simulink subsystem "proc_nav_ros_input"  (R2021a)
settings: Solver=VariableStepAuto  StartTime=0.0  StopTime=10.0  RelTol=1e-3
undefined symbols (not defined in the file): simulink
libraries: robotlib x6, simulink x2
settings Model: Creator=lamarre  LastModifiedBy=lamarre
settings SolverCC: AlgebraicLoopSolver=TrustRegion
settings DebuggingCC: SFMachineParentedDataDiag=warning

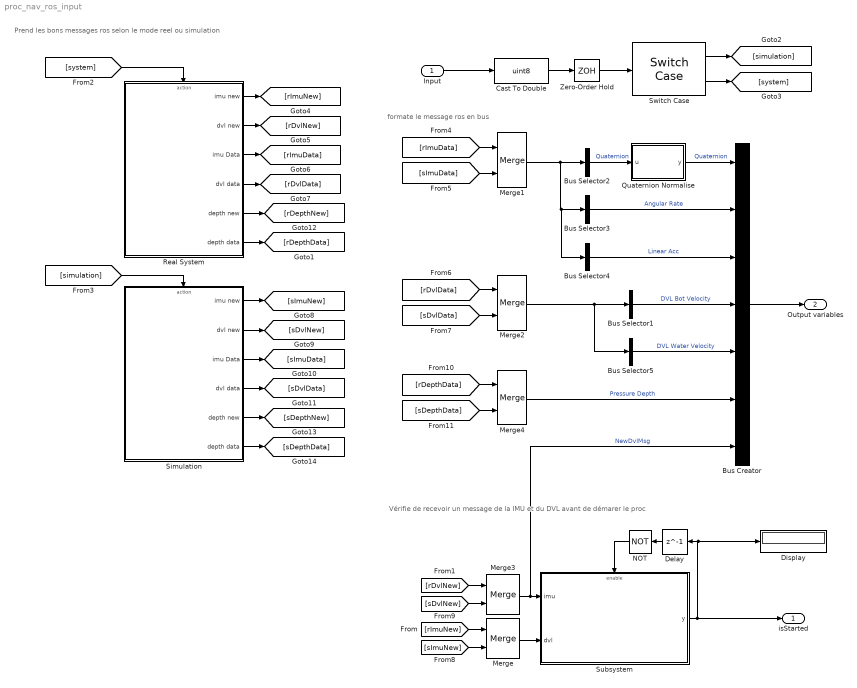
== system proc_nav_ros_input ==
  note: formate le message ros en bus
  note: Prend les bons messages ros selon le mode reel ou simulation
  note: Vérifie de recevoir un message de la IMU et
      |  du DVL avant de démarer le proc
  Input : Inport
  Bus Creator : BusCreator  Inputs=7
  Bus Selector1 : BusSelector  OutputSignals=XVelBtm,YVelBtm,ZVelBtm,EVelBtm  OutputAsBus=on
  Bus Selector2 : BusSelector  OutputSignals=Orientation.W,Orientation.X,Orientation.Y,Orientation.Z  OutputAsBus=on
  Bus Selector3 : BusSelector  OutputSignals=AngularVelocity  OutputAsBus=on
  Bus Selector4 : BusSelector  OutputSignals=LinearAcceleration  OutputAsBus=on
  Bus Selector5 : BusSelector  OutputSignals=Velocity1,Velocity2,Velocity3,Velocity4  OutputAsBus=on
  Cast To Double : DataTypeConversion  OutDataTypeStr=uint8
  Delay : Delay  DelayLength=1  InitialCondition=0
  Display : Display
  Merge{,1..4} (5 alike) : Merge
  NOT : Logic  Operator=NOT  AllPortsSameDT=off  OutDataTypeStr=boolean
  Quaternion Normalise : MATLAB Function  TreatAsAtomicUnit=on
  Real System : Subsystem  TreatAsAtomicUnit=on
  Simulation : Subsystem  TreatAsAtomicUnit=on
  Subsystem : Subsystem
  Switch Case : SwitchCase
  Zero-Order Hold : ZeroOrderHold  SampleTime=simulink.procNav.sampletime
  isStarted : Outport
  Output variables : Outport  Port=2
  wires:
  Bus Selector3/1 -> Bus Creator/2  "Angular Rate"
  Bus Selector1/1 -> Bus Creator/4  "DVL Bot Velocity"
  Bus Creator/1 -> Output variables/1
  Merge1/1 -> Bus Selector2/1, Bus Selector3/1, Bus Selector4/1
  Bus Selector2/1 -> Quaternion Normalise/1(u)  "Quaternion"
  Quaternion Normalise/1(y) -> Bus Creator/1  "Quaternion"
  Bus Selector4/1 -> Bus Creator/3  "Linear Acc"
  Bus Selector5/1 -> Bus Creator/5  "DVL Water Velocity"
  Switch Case/2 -> [system]
  Switch Case/1 -> [simulation]
  [system] -> Real System/Action
  [simulation] -> Simulation/Action
  Zero-Order Hold/1 -> Switch Case/1
  Input/1 -> Cast To Double/1
  Cast To Double/1 -> Zero-Order Hold/1
  Delay/1 -> NOT/1
  NOT/1 -> Subsystem/Enable
  Real System/1(imu new) -> [rImuNew]
  Simulation/4(dvl data) -> [sDvlData]
  Simulation/3(imu Data) -> [sImuData]
  Simulation/2(dvl new) -> [sDvlNew]
  Simulation/1(imu new) -> [sImuNew]
  Real System/4(dvl data) -> [rDvlData]
  Real System/3(imu Data) -> [rImuData]
  Real System/2(dvl new) -> [rDvlNew]
  [rImuData] -> Merge1/1
  [sImuData] -> Merge1/2
  [sDvlData] -> Merge2/2
  [rDvlData] -> Merge2/1
  [rImuNew] -> Merge/1
  [sImuNew] -> Merge/2
  [rDvlNew] -> Merge3/1
  [sDvlNew] -> Merge3/2
  Merge3/1 -> Bus Creator/7, Subsystem/1(imu)  "NewDvlMsg"
  Merge/1 -> Subsystem/2(dvl)
  Merge4/1 -> Bus Creator/6  "Pressure Depth"
  Real System/6(depth data) -> [rDepthData]
  Real System/5(depth new) -> [rDepthNew]
  Simulation/5(depth new) -> [sDepthNew]
  Simulation/6(depth data) -> [sDepthData]
  [sDepthData] -> Merge4/2
  [rDepthData] -> Merge4/1
  Subsystem/1(y) -> isStarted/1, Delay/1, Display/1
  Merge2/1 -> Bus Selector1/1, Bus Selector5/1

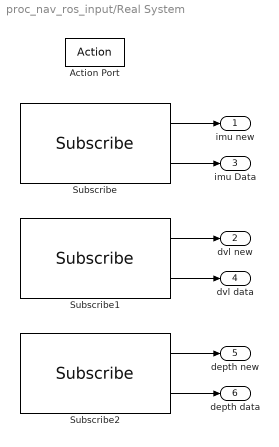
== system proc_nav_ros_input/Real System ==
  Action Port : ActionPort
  Subscribe : robotlib/Subscribe  topicSource=Specify your own  topic=/provider_imu/imu_info  messageType=sensor_msgs/Imu  SampleTime=simulink.procNav.sampletime  legacyBusStruct=off  messageQueueLength=1
  Subscribe1 : robotlib/Subscribe  topicSource=Specify your own  topic=/provider_dvl/dvl_velocity  messageType=sonia_common/BodyVelocityDVL  SampleTime=simulink.procNav.sampletime  legacyBusStruct=off  messageQueueLength=1
  Subscribe2 : robotlib/Subscribe  topicSource=Specify your own  topic=/provider_depth/depth  messageType=std_msgs/Float32  SampleTime=simulink.procNav.sampletime  legacyBusStruct=off  messageQueueLength=1
  imu new : Outport
  dvl new : Outport  Port=2
  imu Data : Outport  Port=3
  dvl data : Outport  Port=4
  depth new : Outport  Port=5
  depth data : Outport  Port=6
  wires:
  Subscribe2/1 -> depth new/1
  Subscribe2/2 -> depth data/1
  Subscribe/2 -> imu Data/1
  Subscribe1/1 -> dvl new/1
  Subscribe1/2 -> dvl data/1
  Subscribe/1 -> imu new/1

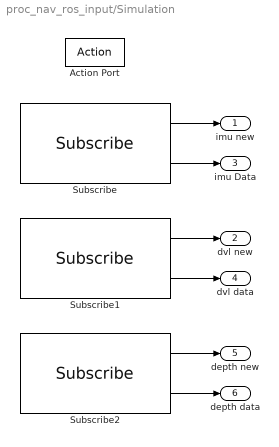
== system proc_nav_ros_input/Simulation ==
  Action Port : ActionPort
  Subscribe : robotlib/Subscribe  topicSource=Specify your own  topic=/proc_simulation/imu_info  messageType=sensor_msgs/Imu  SampleTime=simulink.procNav.sampletime  legacyBusStruct=off  messageQueueLength=1
  Subscribe1 : robotlib/Subscribe  topicSource=Specify your own  topic=/proc_simulation/dvl_velocity  messageType=sonia_common/BodyVelocityDVL  SampleTime=simulink.procNav.sampletime  legacyBusStruct=off  messageQueueLength=1
  Subscribe2 : robotlib/Subscribe  topicSource=Specify your own  topic=/proc_simualtion/depth  messageType=std_msgs/Float32  SampleTime=simulink.procNav.sampletime  legacyBusStruct=off  messageQueueLength=1
  imu new : Outport
  dvl new : Outport  Port=2
  imu Data : Outport  Port=3
  dvl data : Outport  Port=4
  depth new : Outport  Port=5
  depth data : Outport  Port=6
  wires:
  Subscribe2/2 -> depth data/1
  Subscribe2/1 -> depth new/1
  Subscribe/2 -> imu Data/1
  Subscribe1/1 -> dvl new/1
  Subscribe1/2 -> dvl data/1
  Subscribe/1 -> imu new/1

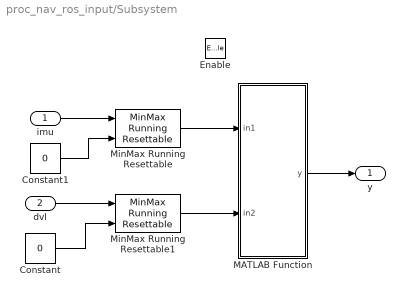
== system proc_nav_ros_input/Subsystem ==
  imu : Inport
  dvl : Inport  Port=2
  Enable : EnablePort
  Constant : Constant  Value=0
  Constant1 : Constant  Value=0
  MATLAB Function : MATLAB Function  TreatAsAtomicUnit=on  SystemSampleTime=simulink.procNav.sampletime
  MinMax Running Resettable : simulink/Math Operations/MinMax Running Resettable  Function=max  vinit=0.0
  MinMax Running Resettable1 : simulink/Math Operations/MinMax Running Resettable  Function=max  vinit=0.0
  y : Outport
  wires:
  Constant1/1 -> MinMax Running Resettable/2
  Constant/1 -> MinMax Running Resettable1/2
  imu/1 -> MinMax Running Resettable/1
  MinMax Running Resettable1/1 -> MATLAB Function/2(in2)
  dvl/1 -> MinMax Running Resettable1/1
  MinMax Running Resettable/1 -> MATLAB Function/1(in1)
  MATLAB Function/1(y) -> y/1

== matlab function proc_nav_ros_input/Quaternion Normalise ==
  data: u input size=4; y output size=4
function y = Normalize(u)
%Normailse le quaternions pour éviter la distortions crée par l'erreur de
% de l'intégration.
d=norm(u);
n=u/d;
if isnan(n)
    y=[1;0;0;0];
else
    y = n;
end

== matlab function proc_nav_ros_input/Subsystem/MATLAB Function ==
  data: in1 input; y output; in2 input
function y = fcn(in1,in2)

if in1+in2 >=2
    y=1;
else
    y=0;
end
